simulink model "simulink_real_estados"  (R2023a)
settings: Solver=VariableStepAuto  StartTime=0.0  StopTime=6  MaxStep=0.001  MinStep=0.0001  RelTol=1e-3  EnableMultiTasking=on
undefined symbols (not defined in the file): Ad, Bd, C, K0d, Kd, Q1, Q2, T
settings Model: Creator=54115  LastModifiedBy=franc
settings SolverCC: AlgebraicLoopSolver=TrustRegion
settings DataIOCC: ReturnWorkspaceOutputs=off
settings OptimizationCC: LifeSpan=inf
settings DebuggingCC: UnconnectedInputMsg=warning  UnconnectedOutputMsg=warning  UnconnectedLineMsg=warning  SFUnexpectedBacktrackingDiag=warning  SFNoUnconditionalDefaultTransitionDiag=warning  ArithmeticOperatorsInVariantConditions=warning
settings ModelReferenceCC: EnableRefExpFcnMdlSchedulingChecks=on
settings SFSimCC: SimUseLocalCustomCode=off  CustomCodeUndefinedFunction=UseInterfaceOnly
settings RTWCC: RTWUseLocalCustomCode=off
settings CodeAppCC: StateflowObjectComments=on
settings GRTTargetCC: TargetLangStandard=C89/C90 (ANSI)
settings ConfigComp: CovMetricSettings=dw  CovSaveCumulativeToWorkspaceVar=on  CovSaveSingleToWorkspaceVar=on  CovExternalEMLEnable=off

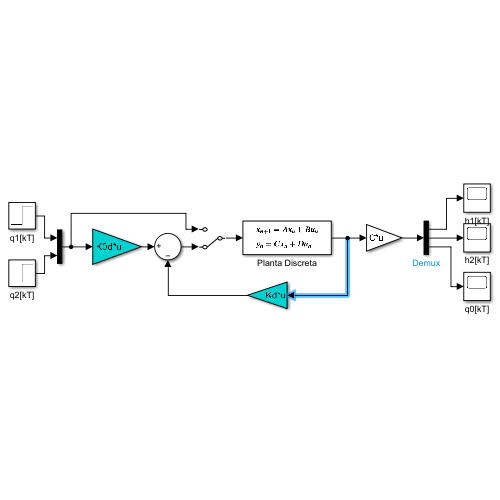
[thumbnail: Simulink's stored preview of the top-level diagram]
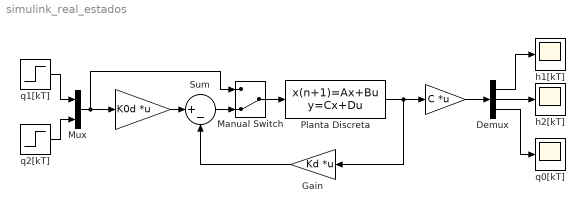
== system simulink_real_estados ==
  " " : Gain  Gain=K0d  Multiplication=Matrix(K*u)
  "   " : Gain  Gain=C  Multiplication=Matrix(K*u)
  Demux : Demux  Outputs=3
  Gain : Gain  Gain=Kd  Multiplication=Matrix(K*u)
  Manual Switch : ManualSwitch  CurrentSetting=0
  Mux : Mux  Inputs=2
  Planta Discreta : DiscreteStateSpace  A=Ad  B=Bd  C=eye(2)  D=zeros(2)  SampleTime=T
  Sum : Sum  Inputs=|+-
  h1[kT] : Scope
  h2[kT] : Scope
  q0[kT] : Scope
  q1[kT] : Step  Time=0  After=Q1  SampleTime=T
  q2[kT] : Step  Time=0  After=Q2  SampleTime=T
  wires:
  Gain/1 -> Sum/2
  " "/1 -> Sum/1
  Planta Discreta/1 -> "   "/1, Gain/1
  Demux/1 -> h1[kT]/1
  Demux/2 -> h2[kT]/1
  Demux/3 -> q0[kT]/1
  q1[kT]/1 -> Mux/1
  q2[kT]/1 -> Mux/2
  Mux/1 -> Manual Switch/1, " "/1
  "   "/1 -> Demux/1
  Sum/1 -> Manual Switch/2
  Manual Switch/1 -> Planta Discreta/1
